simulink model "zad8_obsw"  (R2014b)
settings: Solver=ode45  StartTime=0.0  StopTime=10.0  RelTol=1e-3
values from neighbouring files (symbols this model uses):
  l1 = -(z0+z1)    [zad10.m]    (also in zad9.m = -(z0(i)+z1(i)))
  l2 = z0*z1    [zad10.m]    (also in zad9.m = z0(i)*z1(i))
  Tp = 0.25    [setparam.m]    (also in zad1.m)
settings Model: Creator=kuba  LastModifiedBy=kuba

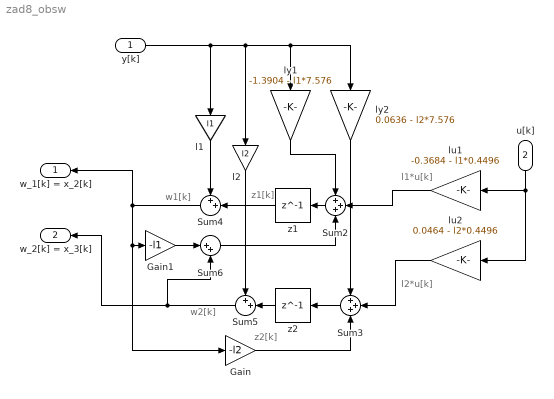
== system zad8_obsw ==
  note: l2*u[k]
  note: l1*u[k]
  note: z2[k]
  note: z1[k]
  note: w1[k]
  note: w2[k]
  y[k] : Inport
  u[k] : Inport  Port=2
  Gain : Gain  Gain=-l2
  Gain1 : Gain  Gain=-l1
  Sum2 : Sum  Inputs=+++
  Sum3 : Sum  Inputs=+++
  Sum4 : Sum  Inputs=++|
  Sum5 : Sum  Inputs=++|
  Sum6 : Sum  Inputs=|++
  l1 : Gain  Gain=l1
  l2 : Gain  Gain=l2
  lu1 : Gain  Gain=-0.3684 - l1*0.4496
  lu2 : Gain  Gain=0.0464 - l2*0.4496
  ly1 : Gain  Gain=-1.3904 - l1*7.576
  ly2 : Gain  Gain=0.0636 - l2*7.576
  z1 : Delay  DelayLength=1  SampleTime=Tp
  z2 : Delay  DelayLength=1  SampleTime=Tp
  w_1[k] = x_2[k] : Outport
  w_2[k] = x_3[k] : Outport  Port=2
  wires:
  u[k]/1 -> lu2/1, lu1/1
  Sum2/1 -> z1/1
  Sum3/1 -> z2/1
  z1/1 -> Sum4/2
  Sum4/1 -> Gain/1, Gain1/1, w_1[k] = x_2[k]/1
  z2/1 -> Sum5/2
  Sum5/1 -> Sum6/2, w_2[k] = x_3[k]/1
  Gain/1 -> Sum3/3
  Gain1/1 -> Sum6/1
  Sum6/1 -> Sum2/3
  lu1/1 -> Sum2/2
  lu2/1 -> Sum3/2
  l1/1 -> Sum4/1
  l2/1 -> Sum5/1
  ly2/1 -> Sum3/1
  ly1/1 -> Sum2/1
  y[k]/1 -> l2/1, ly2/1, ly1/1, l1/1
